simulink model "SimulationANTSMC"  (R2020b)
settings: Solver=ode3  StartTime=0.0  StopTime=100  FixedStep=0.001  RelTol=1e-6  EnableMultiTasking=on
model workspace (MAT data in the model file):
  time = 1
values from neighbouring files (symbols this model uses):
  beta = 2*x(3)/(1+x(3))    [GA_init.m]
  epstar = x(9)    [GA_init.m]
  g0 = x(5)    [GA_init.m]
  g1 = x(6)    [GA_init.m]
  g2 = x(7)    [GA_init.m]
  g3 = x(8)    [GA_init.m]
  gamma = x(3)    [GA_init.m]
  kappa = x(11)    [GA_init.m]
  landa = x(1)    [GA_init.m]
  nu = x(2)    [GA_init.m]
  vu = x(4)    [GA_init.m]
(part 18 of 18)

== matlab function SimulationANTSMC/Subsystem/Uas/MATLAB Function ==
  data: s input; sat output; epstar input
function sat = fcn(s,epstar)

if abs(s)>=epstar
    sat=sign(s);
else
    sat=s./epstar;
    
    end

== matlab function SimulationANTSMC/Subsystem/Uas/MATLAB Function1 ==
  data: s input; psi_dot output; kappa input; vu input
function psi_dot = fcn(s,kappa,vu)
psidot=zeros(6,1);
for i=1:6
    if abs(s(i))>vu
        
        psidot(i)=abs(s(i))/kappa;
        
    else
        
        psidot(i)=0;
    
    end
end

psi_dot=[psidot(1),psidot(2),psidot(3),psidot(4),psidot(5),psidot(6)]';
